simulink model "Helmholtz_LS"  (Simulink 8.0)
settings: Solver=FixedStepDiscrete  StartTime=0.0  StopTime=1.0  FixedStep=1.0  RelTol=1e-3
libraries: Network_library x5
settings Model: Creator=mur  LastModifiedBy=mur
settings DataIOCC: SignalLoggingSaveFormat=ModelDataLogs
settings DebuggingCC: FcnCallInpInsideContextMsg=UseLocalSettings
settings GRTTargetCC: CombineOutputUpdateFcns=off  GRTInterface=on

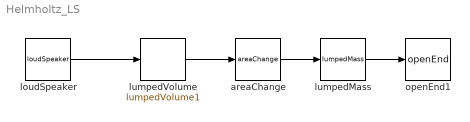
== system Helmholtz_LS ==
  areaChange : Network_library/areaChange  element=areaChange  aj=pi/4*.05^2  D=0
      settings: AttributesFormatString=%<aj> m^2
  loudSpeaker : Network_library/loudSpeaker  element=loudSpeaker  loc=Upstream  Amp=1  c=340  Mach=0.  rho=1.2  D=0  a=1
      settings: AttributesFormatString=%<Amp> m/s
  lumpedMass : Network_library/lumpedMass  element=lumpedMass  Flag=Equivalent length  Leq=1e-2  Veq=1  meq=1e-3
      settings: AttributesFormatString=%<Leq> m
  lumpedVolume : Network_library/lumpedVolume1  element=lumpedVolume  Flag=Equivalent length  Leq=.5  Veq=1
      settings: AttributesFormatString=%<Leq> m
  openEnd1 : Network_library/openEnd  element=openEnd  loc=Downstream  c=100  Mach=0.1  rho=1.2  D=1  a=1
  wires:
  loudSpeaker/1 -> lumpedVolume/1
  lumpedMass/1 -> openEnd1/1
  lumpedVolume/1 -> areaChange/1
  areaChange/1 -> lumpedMass/1
